simulink model "CoVeh_CalcTrqPrpLimErr"  (R2016b)
settings: configuration reference "CodeGenConfigSet" (kept outside this file)
values from neighbouring files (symbols this model uses):
  CoVeh_bLimTboxFenceOut_C = Calibration.Parameter    [init_CoVeh_CalcTrqPrpLimErr.m]
  CoVeh_dtrqLimDwn_C = Calibration.Parameter    [init_CoVeh_CalcTrqPrpLimErr.m]
  CoVeh_dtrqLimUp_C = Calibration.Parameter    [init_CoVeh_CalcTrqPrpLimErr.m]
  CoVeh_trqLim_CUR = Calibration.Parameter    [init_CoVeh_CalcTrqPrpLimErr.m]
  CoVeh_trqLim_CURX = Calibration.Parameter    [init_CoVeh_CalcTrqPrpLimErr.m]
  TRQPRPHIGH_MAX = fi(3000,Trq_Nm)    [init_CoVeh_CalcTrqPrpLimErr.m]
undefined symbols (not defined in the file or in its folder): CoVeh_CalcTrqPrpLimErr_DT
libraries: CXLib x3
settings Model: Creator=Colin  LastModifiedBy=zhoutinglin
settings ConfigSetRef: SourceLocation=Base Workspace

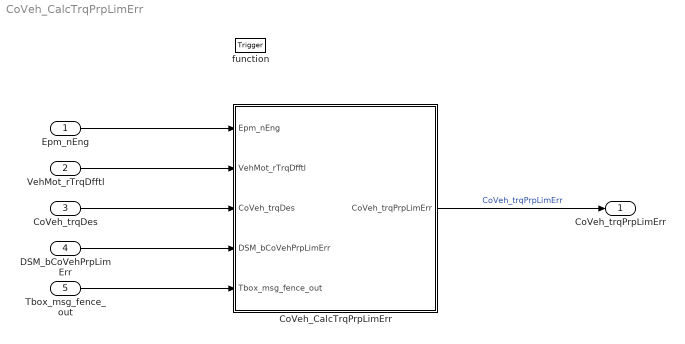
== system CoVeh_CalcTrqPrpLimErr ==
  Epm_nEng : Inport  Tag=rpm  Description=Engine speed  OutMin=0  OutMax=6000  OutDataTypeStr=EngSpeed_rpm
  VehMot_rTrqDfftl : Inport  Description=Torque ratio of differential  Port=2  OutMin=-300  OutMax=300  OutDataTypeStr=TransRatio
  CoVeh_trqDes : Inport  Tag=Nm  Description=Setpoint torque order to the drive train (gearbox output torque)  Port=3  OutMin=-3000  OutMax=3000  OutDataTypeStr=Trq_Nm
  DSM_bCoVehPrpLimErr : Inport  Description=Fault Indicator of System Error on Vehicle Propulsion Torque Limit  Port=4  OutMin=0  OutMax=1  OutDataTypeStr=boolean
  Tbox_msg_fence_out : Inport  Description=fence out message from TBOX  Port=5  OutMin=0  OutMax=255  OutDataTypeStr=uint8
  function : TriggerPort  TriggerType=function-call  VariantControl=Variant
  CoVeh_CalcTrqPrpLimErr : Subsystem
  CoVeh_trqPrpLimErr : Outport  Tag=Nm  Description=limitation torque for propulsion at system error  OutMin=-3000  OutMax=3000  OutDataTypeStr=Trq_Nm
  wires:
  Epm_nEng/1 -> CoVeh_CalcTrqPrpLimErr/1(Epm_nEng)
  VehMot_rTrqDfftl/1 -> CoVeh_CalcTrqPrpLimErr/2(VehMot_rTrqDfftl)
  CoVeh_trqDes/1 -> CoVeh_CalcTrqPrpLimErr/3(CoVeh_trqDes)
  CoVeh_CalcTrqPrpLimErr/1(CoVeh_trqPrpLimErr) -> CoVeh_trqPrpLimErr/1  "CoVeh_trqPrpLimErr"
  DSM_bCoVehPrpLimErr/1 -> CoVeh_CalcTrqPrpLimErr/4(DSM_bCoVehPrpLimErr)
  Tbox_msg_fence_out/1 -> CoVeh_CalcTrqPrpLimErr/5(Tbox_msg_fence_out)

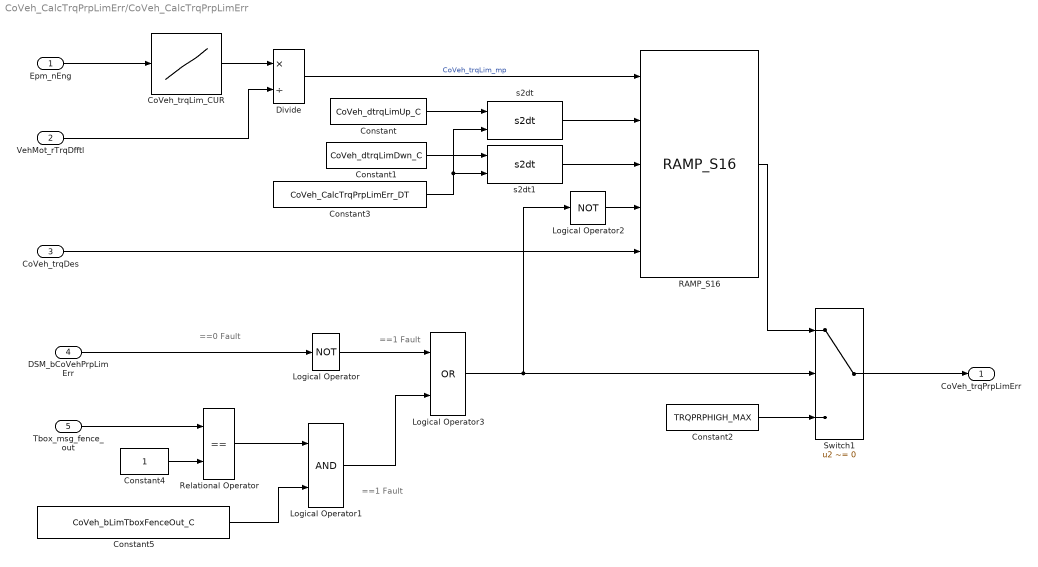
== system CoVeh_CalcTrqPrpLimErr/CoVeh_CalcTrqPrpLimErr ==
  note: ==0 Fault
  note: ==1 Fault
  note: ==1 Fault
  Epm_nEng : Inport  Tag=rpm  Description=Engine speed  OutMin=0  OutMax=6000  OutDataTypeStr=EngSpeed_rpm
  VehMot_rTrqDfftl : Inport  Description=Torque ratio of differential  Port=2  OutMin=-300  OutMax=300  OutDataTypeStr=TransRatio
  CoVeh_trqDes : Inport  Tag=Nm  Description=Setpoint torque order to the drive train (gearbox output torque)  Port=3  OutMin=-3000  OutMax=3000  OutDataTypeStr=Trq_Nm
  DSM_bCoVehPrpLimErr : Inport  Description=Fault Indicator of System Error on Vehicle Propulsion Torque Limit  Port=4  OutDataTypeStr=boolean
  Tbox_msg_fence_out : Inport  Port=5
  CoVeh_trqLim_CUR : Lookup_n-D  NumberOfTableDimensions=1  BreakpointsForDimension1=CoVeh_trqLim_CURX  Table=CoVeh_trqLim_CUR  TableDataTypeStr=Inherit: Inherit from 'Table data'  ExtrapMethod=Clip  InternalRulePriority=Speed  OutDataTypeStr=Inherit: Inherit from 'Table data'  RndMeth=Simplest
  Constant : Constant  Value=CoVeh_dtrqLimUp_C
  Constant1 : Constant  Value=CoVeh_dtrqLimDwn_C
  Constant2 : Constant  Value=TRQPRPHIGH_MAX
  Constant3 : Constant  Value=CoVeh_CalcTrqPrpLimErr_DT
  Constant4 : Constant  OutDataTypeStr=Inherit: Inherit via back propagation
  Constant5 : Constant  Value=CoVeh_bLimTboxFenceOut_C
  Divide : Product  Inputs=*/  OutDataTypeStr=Trq_Nm
  Logical Operator : Logic  Operator=NOT  AllPortsSameDT=off  OutDataTypeStr=boolean
  Logical Operator1 : Logic  AllPortsSameDT=off  OutDataTypeStr=boolean
  Logical Operator2 : Logic  Operator=NOT  AllPortsSameDT=off  OutDataTypeStr=boolean
  Logical Operator3 : Logic  Operator=OR  AllPortsSameDT=off  OutDataTypeStr=boolean
  RAMP_S16 : CXLib/RAMP_S16
  Relational Operator : RelationalOperator  Operator===  OutDataTypeStr=boolean  RndMeth=Simplest
  Switch1 : Switch  Criteria=u2 ~= 0
  s2dt : CXLib/s2dt
  s2dt1 : CXLib/s2dt
  CoVeh_trqPrpLimErr : Outport  Tag=Nm  Description=limitation torque for propulsion at system error  OutMin=-3000  OutMax=3000  OutDataTypeStr=Trq_Nm
  wires:
  Epm_nEng/1 -> CoVeh_trqLim_CUR/1
  CoVeh_trqLim_CUR/1 -> Divide/1
  VehMot_rTrqDfftl/1 -> Divide/2
  Divide/1 -> RAMP_S16/1  "CoVeh_trqLim_mp"
  RAMP_S16/1 -> Switch1/1
  Constant2/1 -> Switch1/3
  Switch1/1 -> CoVeh_trqPrpLimErr/1
  Constant/1 -> s2dt/1
  Constant3/1 -> s2dt1/2, s2dt/2
  Constant1/1 -> s2dt1/1
  s2dt/1 -> RAMP_S16/2
  s2dt1/1 -> RAMP_S16/3
  CoVeh_trqDes/1 -> RAMP_S16/5
  Tbox_msg_fence_out/1 -> Relational Operator/1
  Constant4/1 -> Relational Operator/2
  Relational Operator/1 -> Logical Operator1/1
  Constant5/1 -> Logical Operator1/2
  Logical Operator1/1 -> Logical Operator3/2
  DSM_bCoVehPrpLimErr/1 -> Logical Operator/1
  Logical Operator/1 -> Logical Operator3/1
  Logical Operator3/1 -> Logical Operator2/1, Switch1/2
  Logical Operator2/1 -> RAMP_S16/4
